simulink model "impedance_host"  (R2021b)
settings: Solver=ode1  StartTime=0.0  StopTime=inf  FixedStep=2e-4  RelTol=1e-3
libraries: slrealtimeutilitieslib x1, slrealtimeiplib x1
settings Model: Creator=tcraddoc  LastModifiedBy=wasynczu
settings SolverCC: AlgebraicLoopSolver=TrustRegion
settings DataIOCC: ReturnWorkspaceOutputs=off
settings DebuggingCC: SFMachineParentedDataDiag=warning  ArithmeticOperatorsInVariantConditions=warning
settings SFSimCC: SimUseLocalCustomCode=off  CustomCodeUndefinedFunction=UseInterfaceOnly
settings RTWCC: RTWUseLocalCustomCode=off
settings CodeAppCC: StateflowObjectComments=on

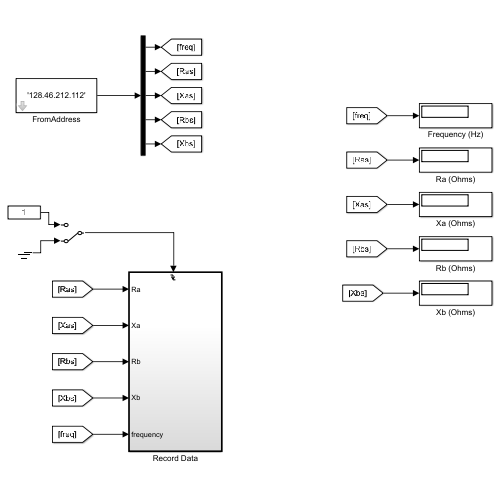
[thumbnail: Simulink's stored preview of the top-level diagram]
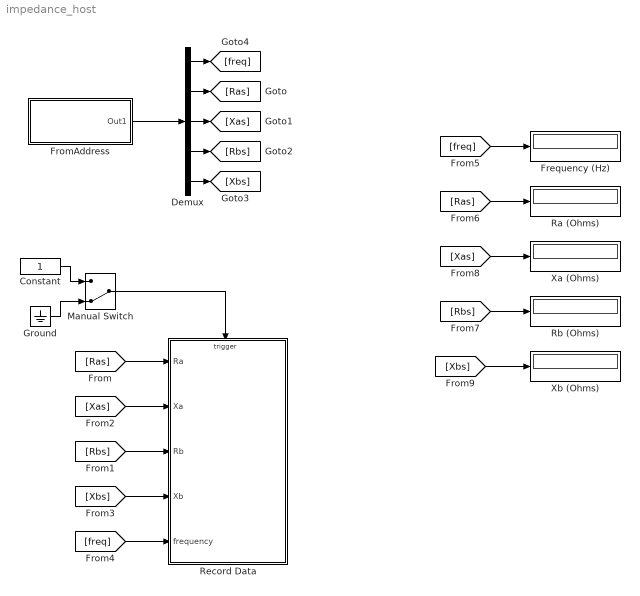
== system impedance_host ==
  Constant : Constant
  Demux : Demux  Outputs=5
  Frequency (Hz) : Display
  FromAddress : Subsystem  mask{fromIPAddress='128.46.212.112'}
      mask prompts: fromIPAddress "From IP Address"
      mask Display: disp((get_param(gcb,'fromIPAddress')))
  Ground : Ground
  Manual Switch : ManualSwitch  CurrentSetting=0
  Ra (Ohms) : Display
  Rb (Ohms) : Display
  Record Data : Subsystem  TreatAsAtomicUnit=on
  Xa (Ohms) : Display
  Xb (Ohms) : Display
  wires:
  [Ras] -> Ra (Ohms)/1
  [Xas] -> Xa (Ohms)/1
  [Xbs] -> Xb (Ohms)/1
  [Ras] -> Record Data/1(Ra)
  [Rbs] -> Record Data/3(Rb)
  [Xas] -> Record Data/2(Xa)
  [Xbs] -> Record Data/4(Xb)
  [freq] -> Record Data/5(frequency)
  Ground/1 -> Manual Switch/2
  Constant/1 -> Manual Switch/1
  Manual Switch/1 -> Record Data/Trigger
  FromAddress/1(Out1) -> Demux/1
  Demux/1 -> [freq]
  Demux/3 -> [Xas]
  Demux/2 -> [Ras]
  Demux/4 -> [Rbs]
  Demux/5 -> [Xbs]
  [freq] -> Frequency (Hz)/1
  [Rbs] -> Rb (Ohms)/1

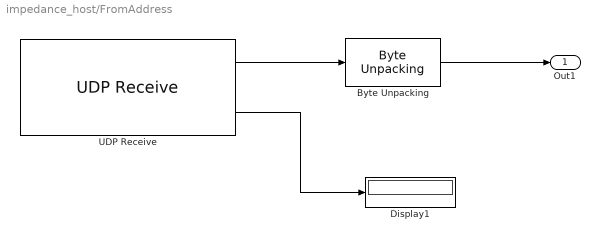
== system impedance_host/FromAddress ==
  Byte Unpacking : slrealtimeutilitieslib/Byte Unpacking  MaskUnpackedDataTypes={['double']}  MaskUnpackedDataSizes={[5]}  MaskAlignment=1
      settings: SourceProductBaseCode=XP
  Display1 : Display
  UDP Receive : slrealtimeiplib/UDP Receive  useHostTargetConn=on  ipAddress=128.46.212.188  localPort=34  rcvWidth=40  rcvFmAny=off  fmAddress=fromIPAddress  sampleTime=1e-3
      settings: SourceProductBaseCode=XP
  Out1 : Outport
  wires:
  Byte Unpacking/1 -> Out1/1
  UDP Receive/2 -> Display1/1
  UDP Receive/1 -> Byte Unpacking/1

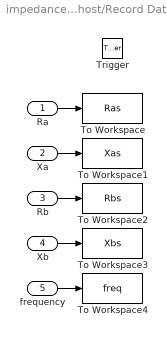
== system impedance_host/Record Data ==
  Ra : Inport
  Xa : Inport  Port=2
  Rb : Inport  Port=3
  Xb : Inport  Port=4
  frequency : Inport  Port=5
  Trigger : TriggerPort  TriggerType=falling  VariantControl=Variant
  To Workspace : ToWorkspace  VariableName=Ras  SampleTime=-1
  To Workspace1 : ToWorkspace  VariableName=Xas  SampleTime=-1
  To Workspace2 : ToWorkspace  VariableName=Rbs  SampleTime=-1
      settings: Save2DSignal=2-D array (concatenate along first dimension)
  To Workspace3 : ToWorkspace  VariableName=Xbs  SampleTime=-1
  To Workspace4 : ToWorkspace  VariableName=freq  SampleTime=-1
      settings: Save2DSignal=2-D array (concatenate along first dimension)
  wires:
  Ra/1 -> To Workspace/1
  Xa/1 -> To Workspace1/1
  Rb/1 -> To Workspace2/1
  Xb/1 -> To Workspace3/1
  frequency/1 -> To Workspace4/1
